simulink model "LQR_vehicle_dynamic_model"  (R2021b)
settings: Solver=ode45  StartTime=0.0  StopTime=60  RelTol=0.1
model workspace (MAT data in the model file):
  k1 = [0.316227766019 0.316227766017 0.316227766017 0.316227766017 0.316227766017 0.316227766017 0.316227766017 0.316227766017 0.316227766017 0.316227766017 0.316227766017 0.316227766017 ... (5000 elements, 1x5000)]
  k2 = [0.000301883202587 0.000603764374018 0.000905641483218 0.00120751249925 0.00150937539142 0.00181122812931 0.00211306868289 0.00241489502258 0.00271670511931 0.00301849694462 0.00332026847071 0.00362201767054 ... (5000 elements, 1x5000)]
  k3 = [0.945396449835 0.945404346198 0.945417506418 0.945435929946 0.945459615988 0.945488563526 0.945522771323 0.945562237918 0.945606961617 0.945656940508 0.945712172453 0.945772655093 ... (5000 elements, 1x5000)]
  k4 = [0.000322785568317 0.000645569647506 0.000968350748438 0.00129112738198 0.00161389805896 0.00193666129021 0.00225941558652 0.00258215945866 0.00290489141734 0.00322760997326 0.00355031363705 0.00387300091929 ... (5000 elements, 1x5000)]
  kappar = [0 0 0 0 0 0 0 0 0 0 0 0 ... (4802 elements, 1x4802)]
  thetar = [0 0 0 0 0 0 0 0 0 0 0 0 ... (4802 elements, 1x4802)]
  xr = [0.0501253132832 0.100250626566 0.15037593985 0.200501253133 0.250626566416 0.300751879699 0.350877192982 0.401002506266 0.451127819549 0.501253132832 0.551378446115 0.601503759398 ... (4802 elements, 1x4802)]
  yr = [0 0 0 0 0 0 0 0 0 0 0 0 ... (4802 elements, 1x4802)]
libraries: simulink x1
(part 2 of 2)

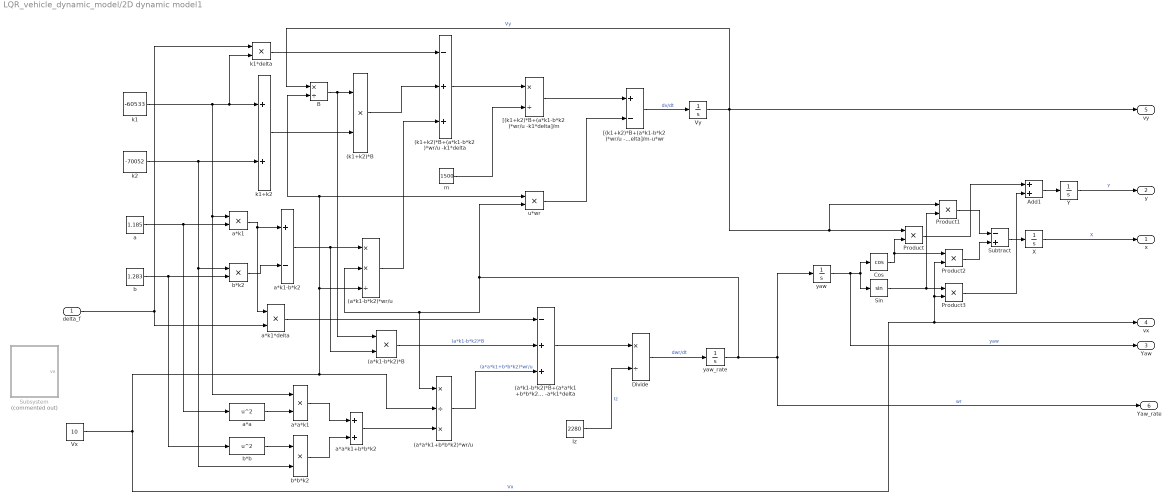
== system LQR_vehicle_dynamic_model/2D dynamic model1 ==
  delta_f : Inport
  (a*a*k1+b*b*k2)*wr/u : Product  Inputs=*/*
  (a*k1-b*k2)*B : Product
  (a*k1-b*k2)*B+(a*a*k1+b*b*k2)*wr/u -a*k1*delta : Sum  Inputs=-++
  (a*k1-b*k2)*wr/u : Product  Inputs=**/
  (k1+k2)*B : Product
  (k1+k2)*B+(a*k1-b*k2)*wr/u -k1*delta : Sum  Inputs=-++
  Add1 : Sum
  B : Product  Inputs=*/
  Cos : Trigonometry  Operator=cos
  Divide : Product  Inputs=*/
  Iz : Constant  Value=2280
  Product{,1..3} (4 alike) : Product
  Sin : Trigonometry
  Subsystem : Subsystem  Commented=on
  Subtract : Sum  Inputs=-+
  Vx : Constant  Value=10
  Vy : Integrator
  X : Integrator
  Y : Integrator
  "[(k1+k2)*B+(a*k1-b*k2)*wr/u -k1*delta]/m" : Product  Inputs=*/
  "[(k1+k2)*B+(a*k1-b*k2)*wr/u -k1*delta]/m-u*wr" : Sum  Inputs=+-
  a : Constant  Value=1.185
  a*a : Fcn  Expr=u^2
  a*a*k1 : Product
  a*a*k1+b*b*k2 : Sum
  a*k1 : Product
  a*k1*delta : Product
  a*k1-b*k2 : Sum  Inputs=+-
  b : Constant  Value=1.283
  b*b : Fcn  Expr=u^2
  b*b*k2 : Product
  b*k2 : Product
  k1 : Constant  Value=-60533
  k1*delta : Product
  k1+k2 : Sum
  k2 : Constant  Value=-70052
  m : Constant  Value=1500
  u*wr : Product
  yaw : Integrator
  yaw_rate : Integrator
  x : Outport  VectorParamsAs1DForOutWhenUnconnected=off
  y : Outport  Port=2  VectorParamsAs1DForOutWhenUnconnected=off
  Yaw : Outport  Port=3  VectorParamsAs1DForOutWhenUnconnected=off
  vx : Outport  Port=4  VectorParamsAs1DForOutWhenUnconnected=off
  vy : Outport  Port=5  VectorParamsAs1DForOutWhenUnconnected=off
  Yaw_rate : Outport  Port=6  VectorParamsAs1DForOutWhenUnconnected=off
  wires:
  (a*a*k1+b*b*k2)*wr/u/1 -> (a*k1-b*k2)*B+(a*a*k1+b*b*k2)*wr/u -a*k1*delta/3  "(a*a*k1+b*b*k2)*wr/u"
  b/1 -> b*k2/2, b*b/1
  (a*k1-b*k2)*B+(a*a*k1+b*b*k2)*wr/u -a*k1*delta/1 -> Divide/1
  k1+k2/1 -> (k1+k2)*B/2
  yaw/1 -> Yaw/1, Cos/1, Sin/1  "yaw"
  k1/1 -> k1*delta/2, k1+k2/1, a*a*k1/1, a*k1/1
  k2/1 -> k1+k2/2, b*b*k2/2, b*k2/1
  b*b/1 -> b*b*k2/1
  Product2/1 -> Subtract/2
  B/1 -> (a*k1-b*k2)*B/1, (k1+k2)*B/1
  Add1/1 -> Y/1
  Sin/1 -> Product3/1, Product1/2
  "[(k1+k2)*B+(a*k1-b*k2)*wr/u -k1*delta]/m"/1 -> "[(k1+k2)*B+(a*k1-b*k2)*wr/u -k1*delta]/m-u*wr"/1
  yaw_rate/1 -> (a*k1-b*k2)*wr/u/2, (a*a*k1+b*b*k2)*wr/u/1, u*wr/2, yaw/1, Yaw_rate/1  "wr"
  a/1 -> a*k1/2, a*a/1
  Product/1 -> Add1/1
  a*k1-b*k2/1 -> (a*k1-b*k2)*B/2, (a*k1-b*k2)*wr/u/1
  Product3/1 -> Add1/2
  b*b*k2/1 -> a*a*k1+b*b*k2/2
  Vy/1 -> vy/1, Product/1, Product1/1, B/1  "Vy"
  a*a*k1/1 -> a*a*k1+b*b*k2/1
  "[(k1+k2)*B+(a*k1-b*k2)*wr/u -k1*delta]/m-u*wr"/1 -> Vy/1  "dv/dt"
  u*wr/1 -> "[(k1+k2)*B+(a*k1-b*k2)*wr/u -k1*delta]/m-u*wr"/2
  (k1+k2)*B+(a*k1-b*k2)*wr/u -k1*delta/1 -> "[(k1+k2)*B+(a*k1-b*k2)*wr/u -k1*delta]/m"/1
  a*k1/1 -> a*k1*delta/1, a*k1-b*k2/1
  a*a*k1+b*b*k2/1 -> (a*a*k1+b*b*k2)*wr/u/3
  Iz/1 -> Divide/2  "Iz"
  (a*k1-b*k2)*B/1 -> (a*k1-b*k2)*B+(a*a*k1+b*b*k2)*wr/u -a*k1*delta/2  "(a*k1-b*k2)*B"
  (a*k1-b*k2)*wr/u/1 -> (k1+k2)*B+(a*k1-b*k2)*wr/u -k1*delta/3
  Vx/1 -> B/2, u*wr/1, (a*k1-b*k2)*wr/u/3, (a*a*k1+b*b*k2)*wr/u/2, vx/1, Product3/2, Product2/2  "Vx"
  delta_f/1 -> a*k1*delta/2, k1*delta/1
  a*a/1 -> a*a*k1/2
  Y/1 -> y/1  "Y"
  (k1+k2)*B/1 -> (k1+k2)*B+(a*k1-b*k2)*wr/u -k1*delta/2
  Cos/1 -> Product2/1, Product/2
  a*k1*delta/1 -> (a*k1-b*k2)*B+(a*a*k1+b*b*k2)*wr/u -a*k1*delta/1
  b*k2/1 -> a*k1-b*k2/2
  k1*delta/1 -> (k1+k2)*B+(a*k1-b*k2)*wr/u -k1*delta/1
  m/1 -> "[(k1+k2)*B+(a*k1-b*k2)*wr/u -k1*delta]/m"/2
  Divide/1 -> yaw_rate/1  "dwr/dt"
  Subtract/1 -> X/1
  Product1/1 -> Subtract/1
  X/1 -> x/1  "X"

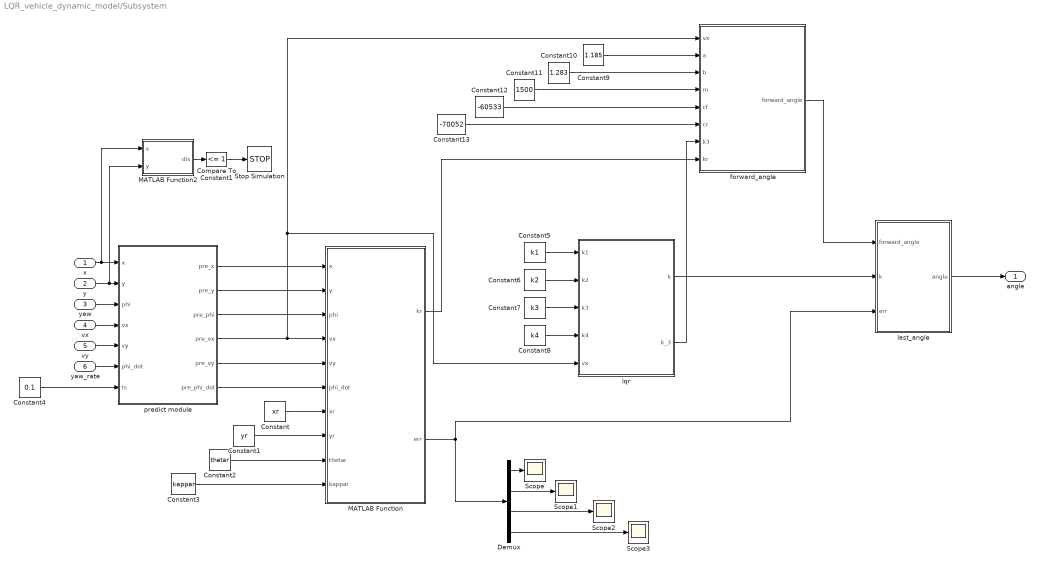
== system LQR_vehicle_dynamic_model/Subsystem ==
  x : Inport
  y : Inport  Port=2
  yaw : Inport  Port=3
  vx : Inport  Port=4
  vy : Inport  Port=5
  yaw_rate : Inport  Port=6
  Compare To Constant1 : simulink/Logic and Bit Operations/Compare To Constant  relop=<=  const=1  OutDataTypeStr=boolean
  Constant : Constant  Value=xr
  Constant1 : Constant  Value=yr
  Constant10 : Constant  Value=1.283
  Constant11 : Constant  Value=1500
  Constant12 : Constant  Value=-60533
  Constant13 : Constant  Value=-70052
  Constant2 : Constant  Value=thetar
  Constant3 : Constant  Value=kappar
  Constant4 : Constant  Value=0.1
  Constant5 : Constant  Value=k1
  Constant6 : Constant  Value=k2
  Constant7 : Constant  Value=k3
  Constant8 : Constant  Value=k4
  Constant9 : Constant  Value=1.185
  Demux : Demux
  MATLAB Function : MATLAB Function  TreatAsAtomicUnit=on
  MATLAB Function2 : MATLAB Function  TreatAsAtomicUnit=on
  Scope{,1..3} (4 alike) : Scope
  Stop Simulation : Stop
  forward_angle : MATLAB Function  TreatAsAtomicUnit=on
  last_angle : MATLAB Function  TreatAsAtomicUnit=on
  lqr : MATLAB Function  TreatAsAtomicUnit=on
  predict module : MATLAB Function  TreatAsAtomicUnit=on
  angle : Outport
  wires:
  Demux/3 -> Scope2/1
  Demux/4 -> Scope3/1
  Constant/1 -> MATLAB Function/7(xr)
  Demux/2 -> Scope1/1
  MATLAB Function/2(err) -> last_angle/3(err), Demux/1
  Constant3/1 -> MATLAB Function/10(kappar)
  Constant2/1 -> MATLAB Function/9(thetar)
  Constant1/1 -> MATLAB Function/8(yr)
  Demux/1 -> Scope/1
  x/1 -> predict module/1(x), MATLAB Function2/1(x)
  y/1 -> MATLAB Function2/2(y), predict module/2(y)
  yaw/1 -> predict module/3(phi)
  vx/1 -> predict module/4(vx)
  vy/1 -> predict module/5(vy)
  yaw_rate/1 -> predict module/6(phi_dot)
  Constant4/1 -> predict module/7(ts)
  predict module/1(pre_x) -> MATLAB Function/1(x)
  predict module/2(pre_y) -> MATLAB Function/2(y)
  predict module/3(pre_phi) -> MATLAB Function/3(phi)
  predict module/4(pre_vx) -> forward_angle/1(vx), lqr/5(vx), MATLAB Function/4(vx)
  predict module/5(pre_vy) -> MATLAB Function/5(vy)
  predict module/6(pre_phi_dot) -> MATLAB Function/6(phi_dot)
  Constant5/1 -> lqr/1(k1)
  Constant6/1 -> lqr/2(k2)
  Constant7/1 -> lqr/3(k3)
  Constant8/1 -> lqr/4(k4)
  MATLAB Function/1(kr) -> forward_angle/8(kr)
  Constant9/1 -> forward_angle/2(a)
  Constant10/1 -> forward_angle/3(b)
  Constant11/1 -> forward_angle/4(m)
  Constant12/1 -> forward_angle/5(cf)
  Constant13/1 -> forward_angle/6(cr)
  forward_angle/1(forward_angle) -> last_angle/1(forward_angle)
  lqr/1(k) -> last_angle/2(k)
  last_angle/1(angle) -> angle/1
  Compare To Constant1/1 -> Stop Simulation/1
  MATLAB Function2/1(dis) -> Compare To Constant1/1
  lqr/2(k_3) -> forward_angle/7(k3)

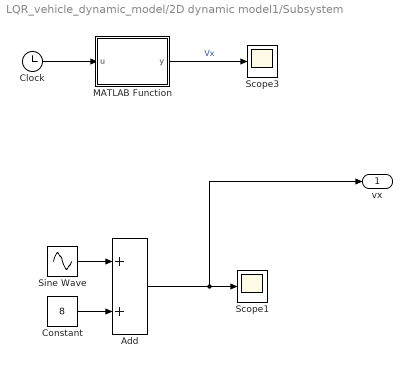
== system LQR_vehicle_dynamic_model/2D dynamic model1/Subsystem ==
  Add : Sum
  Clock : Clock
  Constant : Constant  Value=8
  MATLAB Function : MATLAB Function  TreatAsAtomicUnit=on
  Scope1 : Scope
  Scope3 : Scope
  Sine Wave : Sin  Amplitude=5  Frequency=0.05*pi  SampleTime=0.1
  vx : Outport
  wires:
  MATLAB Function/1(y) -> Scope3/1  "Vx"
  Sine Wave/1 -> Add/1
  Clock/1 -> MATLAB Function/1(u)
  Add/1 -> vx/1, Scope1/1
  Constant/1 -> Add/2

== matlab function LQR_vehicle_dynamic_model/Subsystem/predict module ==
  data: x input; pre_x output; y input; phi input; vx input; vy input; phi_dot input; ts input; pre_y output; pre_phi output; pre_vx output; pre_vy output; pre_phi_dot output
function [pre_x,pre_y,pre_phi,pre_vx,pre_vy,pre_phi_dot] = fcn(x,y,phi,vx,vy,phi_dot,ts)
pre_x=x+vx*ts*cos(phi)-vy*ts*sin(phi);
pre_y=y+vy*ts*cos(phi)+vx*ts*sin(phi);
pre_phi=phi+phi_dot*ts;
pre_vx=vx;
pre_vy=vy;
pre_phi_dot=phi_dot;
end

== matlab function LQR_vehicle_dynamic_model/Subsystem/MATLAB Function ==
  data: x input; kr output; y input; phi input; vx input; vy input; phi_dot input; xr input; yr input; thetar input; kappar input; err output
function [kr,err] = fcn(x,y,phi,vx,vy,phi_dot,xr,yr,thetar,kappar)
n=length(xr);
d_min=(x-xr(1))^2+(y-yr(1))^2;
min=1;
for i=1:n
    d=(x-xr(i))^2+(y-yr(i))^2;
    if d<d_min
        d_min=d;
        min=i;
    end
end
dmin=min;
tor=[cos(thetar(dmin));sin(thetar(dmin))];
nor=[-sin(thetar(dmin));cos(thetar(dmin))];
d_err=[x-xr(dmin);y-yr(dmin)];
ed=nor'*d_err;
es=tor'*d_err;
%projection_point_thetar=thetar(dmin);   %apollo
projection_point_thetar=thetar(dmin)+kappar(dmin)*es;
ed_dot=vy*cos(phi-projection_point_thetar)+vx*sin(phi-projection_point_thetar);
ephi=sin(phi-projection_point_thetar);
s_dot=vx*cos(phi-projection_point_thetar)-vy*sin(phi-projection_point_thetar);
s_dot=s_dot/(1-kappar(dmin)*ed);
ephi_dot=phi_dot-kappar(dmin)*s_dot;
kr=kappar(dmin);
err=[ed;ed_dot;ephi;ephi_dot];
end

== matlab function LQR_vehicle_dynamic_model/Subsystem/lqr ==
  data: k1 input; k2 input; k3 input; k4 input; vx input; k output; k_3 output
function [k,k_3] = fcn(k1,k2,k3,k4,vx)
if abs(vx)<0.01
    k=[0,0,0,0];
    k_3 = 0;
else
    index=round(vx/0.01);   %四舍五入的函数
    k=[k1(index),k2(index),k3(index),k4(index)];
    k_3 = k3(index);
end
end

== matlab function LQR_vehicle_dynamic_model/Subsystem/forward_angle ==
  data: vx input; forward_angle output; a input; b input; m input; cf input; cr input; k3 input; kr input
function forward_angle = fcn(vx,a,b,m,cf,cr,k3,kr)

forward_angle=kr*(a+b-b*k3-(m*vx*vx/(a+b))*((b/cf)+(a/cr)*k3-a/(cr)));

end

== matlab function LQR_vehicle_dynamic_model/Subsystem/last_angle ==
  data: forward_angle input; angle output; k input; err input
function angle = fcn(forward_angle,k,err)

angle=-k*err+forward_angle;
 
end

== matlab function LQR_vehicle_dynamic_model/2D dynamic model1/Subsystem/MATLAB Function ==
  data: u input; y output
function y = fcn(u)

if u <= 25
    y = 5+0.2*u;
else
    y = 10;
end

== matlab function LQR_vehicle_dynamic_model/Subsystem/MATLAB Function2 ==
  data: x input; dis output; y input
function dis = fcn(x, y)

x0 = 240;
y0 = 0;
dis = ((x-x0)^2 + (y-y0)^2)^0.5;

end
